simulink library "Lib_TurboC_FlowStart_TMATSC"  (R2019b)
settings: Solver=ode45  StartTime=0.0  StopTime=10.0  RelTol=1e-3  EnableMultiTasking=on
Description:
  | Thomas Modules
settings Model: Creator=jwchapm2  LastModifiedBy=bhisma
settings DataIOCC: LimitDataPoints=on  SaveFormat=Array  ReturnWorkspaceOutputs=off
settings OptimizationCC: ExpressionDepthLimit=2147483647  LifeSpan=inf
settings DebuggingCC: UnderspecifiedInitializationDetection=Classic  MergeDetectMultiDrivingBlocksExec=none  SolverPrmCheckMsg=warning  StateNameClashWarn=warning  SFUnexpectedBacktrackingDiag=warning  SFNoUnconditionalDefaultTransitionDiag=warning  SFExecutionAtInitializationDiag=none  ArithmeticOperatorsInVariantConditions=warning
settings HardwareCC: ProdBitPerPointer=32  ProdBitPerSizeT=32  ProdBitPerPtrDiffT=32  ProdLargestAtomicFloat=None  ProdIntDivRoundTo=Undefined  ProdEndianess=Unspecified  ProdWordSize=32  ProdHWDeviceType=32-bit Generic
settings ModelReferenceCC: PropagateSignalLabelsOutOfModel=off
settings SFSimCC: SimUseLocalCustomCode=off  CustomCodeUndefinedFunction=UseInterfaceOnly
settings RTWCC: RTWUseLocalCustomCode=off
settings CodeAppCC: StateflowObjectComments=on
settings GRTTargetCC: TargetLangStandard=C89/C90 (ANSI)  GeneratePreprocessorConditionals=Disable all
settings ConfigComp: CovMetricSettings=dw  CovHtmlReporting=on  CovSaveCumulativeToWorkspaceVar=on  CovSaveSingleToWorkspaceVar=on  CovExternalEMLEnable=off  CovSFcnEnable=off

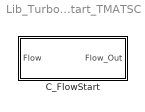
== system Lib_TurboC_FlowStart_TMATSC ==
  C_FlowStart : Subsystem  mask(TMATS: Flow Start Library Block, cantera){Tt_M=518.17, Pt_M=14.696, comp1_M=1, comp2_M=0, comp3_M=0, comp4_M=0, comp5_M=0, comp6_M=0}
      mask prompts: Tt_M "Tt_M - Exit Temperature [R]"; Pt_M "Pt_M - Exit Pressure[psia]"; comp1_M "comp1_M - species 1 [weight frac]"; comp2_M "comp2_M - species 2 [weight frac]"; comp3_M "comp3_M - species 3 [weight frac]"; comp4_M "comp4_M - species 4 [weight frac]"; comp5_M "comp5_M - species 5 [weight frac]"; comp6_M "comp6_M - species 6 [weight frac]"
      mask help:
      | The flow start block creates a T-MATS cantera formated flow from specified inputs. Flow composition definitions below relate to the proportional of the species by weight. Species definitions are located with the catneraload.m file.
      | This block makes use of the Cantera software package.
      mask Help: web(which('TurboC_TMATSC_FS.html'),'-helpbrowser')
      mask Display:
      | color('blue'); port_label('input',1,'Flow')
      | color('blue'); port_label('output',1,'Flow Out')

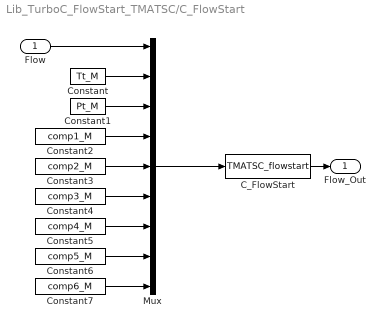
== system Lib_TurboC_FlowStart_TMATSC/C_FlowStart ==
  Flow : Inport
  C_FlowStart : M-S-Function  FunctionName=TMATSC_flowstart
  Constant : Constant  Value=Tt_M
  Constant1 : Constant  Value=Pt_M
  Constant2 : Constant  Value=comp1_M
  Constant3 : Constant  Value=comp2_M
  Constant4 : Constant  Value=comp3_M
  Constant5 : Constant  Value=comp4_M
  Constant6 : Constant  Value=comp5_M
  Constant7 : Constant  Value=comp6_M
  Mux : Mux  Inputs=9
  Flow_Out : Outport
  wires:
  C_FlowStart/1 -> Flow_Out/1
  Flow/1 -> Mux/1
  Mux/1 -> C_FlowStart/1
  Constant/1 -> Mux/2
  Constant1/1 -> Mux/3
  Constant2/1 -> Mux/4
  Constant3/1 -> Mux/5
  Constant4/1 -> Mux/6
  Constant5/1 -> Mux/7
  Constant6/1 -> Mux/8
  Constant7/1 -> Mux/9
